simulink model "FBL_InvPD_RL"  (R2024b)
settings: Solver=VariableStepAuto  StartTime=0.0  StopTime=12  RelTol=1e-3
libraries: slpidlib x2, rllib x1
settings Model: Creator=shree  LastModifiedBy=shree

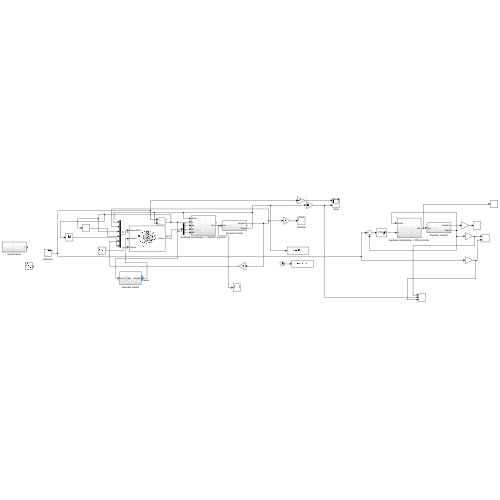
[thumbnail: Simulink's stored preview of the top-level diagram]
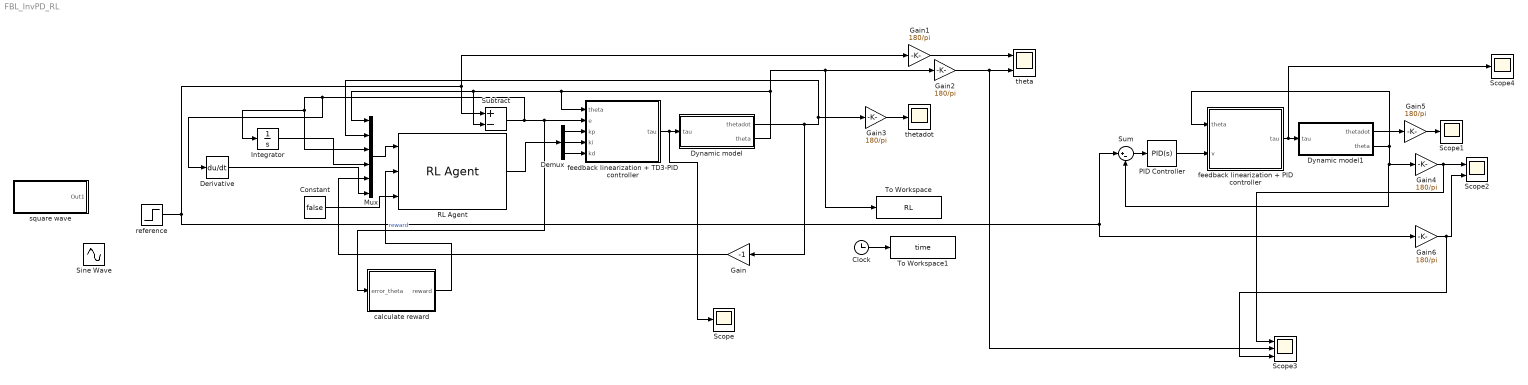
== system FBL_InvPD_RL ==
  Clock : Clock
  Constant : Constant  Value=false
  Demux : Demux  Outputs=3
  Derivative : Derivative
  Dynamic model : Subsystem
  Dynamic model1 : Subsystem
  Gain : Gain  Gain=-1
  Gain{1..6} (6 alike) : Gain  Gain=180/pi
  Integrator : Integrator
  Mux : Mux  Inputs=6
  PID Controller : slpidlib/PID Controller  Controller=PID  Form=Parallel  TimeDomain=Continuous-time  UseExternalTs=off  SampleTime=-1  IntegratorMethod=Forward Euler  FilterMethod=Forward Euler  ControllerParametersSource=internal  P=5.32832873411681  I=1.90556460171503  UseKiTs=off  D=3.52131946383864  UseExternalDerivativeSource=off  N=800  UseFilter=on  TunerSelectOption=Transfer Function Based (PID Tuner App)  InitialConditionSource=internal  InitialConditionForIntegrator=0  InitialConditionForFilter=0  DifferentiatorICPrevScaledInput=0  ExternalReset=none  TrackingMode=off  Kt=1  LimitOutput=on  SatLimitsSource=internal  UpperSaturationLimit=30  LowerSaturationLimit=-30  LinearizeAsGain=on  AntiWindupMode=none  Kb=1  LimitIntegrator=off  UpperIntegratorSaturationLimit=inf  LowerIntegratorSaturationLimit=-inf  POutMin=[]  POutMax=[]  IOutMin=[]  IOutMax=[]  DOutMin=[]  DOutMax=[]  NOutMin=[]  NOutMax=[]  SumOutMin=[]  SumOutMax=[]  SaturationOutMin=[]  SaturationOutMax=[]  PParamMin=[]  PParamMax=[]  IParamMin=[]  IParamMax=[]  DParamMin=[]  DParamMax=[]  NParamMin=[]  NParamMax=[]  KbParamMin=[]  KbParamMax=[]  KtParamMin=[]  KtParamMax=[]  KbOutMin=[]  KbOutMax=[]  KtOutMin=[]  KtOutMax=[]  IntegratorOutMin=[]  IntegratorOutMax=[]  FilterOutMin=[]  FilterOutMax=[]  SumI1OutMin=[]  SumI1OutMax=[]  SumI2OutMin=[]  SumI2OutMax=[]  SumI3OutMin=[]  SumI3OutMax=[]  SumI4OutMin=[]  SumI4OutMax=[]  SumDOutMin=[]  SumDOutMax=[]  DifferentiatorOutMin=[]  DifferentiatorOutMax=[]  FilterDiffOutCoefMin=[]  FilterDiffOutCoefMax=[]  ReciprocalOutMin=[]  ReciprocalOutMax=[]  SumDenOutMin=[]  SumDenOutMax=[]  SumNumOutMin=[]  SumNumOutMax=[]  DivideOutMin=[]  DivideOutMax=[]  UdiffTsProdOutMin=[]  UdiffTsProdOutMax=[]  NTsProdOutMin=[]  NTsProdOutMax=[]  UintegralTsProdOutMin=[]  UintegralTsProdOutMax=[]  UngainTsProdOutMin=[]  UngainTsProdOutMax=[]  ClampingZeroOutDataTypeStr=Inherit: Inherit via back propagation  ClampingZeroOutMin=[]  ClampingZeroOutMax=[]  FilterDenConstantOutDataTypeStr=Inherit: Inherit via back propagation  FilterDenConstantOutMin=[]  FilterDenConstantOutMax=[]  PCopyOutDataTypeStr=Inherit: Inherit via back propagation  PCopyOutMin=[]  PCopyOutMax=[]  NCopyOutDataTypeStr=Inherit: Inherit via back propagation  NCopyOutMin=[]  NCopyOutMax=[]  IntegratorContinuousStateAttributes=''  IntegratorStateMustResolveToSignalObject=off  IntegratorRTWStateStorageClass=Auto  FilterContinuousStateAttributes=''  FilterStateMustResolveToSignalObject=off  FilterRTWStateStorageClass=Auto  ParallelPVariant=InternalParameters  IdealPVariant=Disabled  IVariant=InternalParameters  DVariant=InternalParameters  IntegratorVariant=Continuous  SatVariant=Enabled  AWVariant=Passthrough  PCopyVariant=Disabled  TRVariant=Disabled  FdbkBlocksVariant=Forward  IdealPFdbkVariant=Disabled  SatFdbkVariant=Disabled  DerivativeFilterVariant=ContFilter  NVariant=InternalParameters  NCopyVariant=Disabled  FilterICVariant=InternalICsFilter  IntegratorICVariant=InternalICs  ExternalResetVariant=Disabled  TRSumVariant=Passthrough  SumFdbkVariant=Disabled  SumVariant=Sum_PID  TsampFilterVariant=InternalTs  TsampNgainVariant=Passthrough  TsampIntegralVariant=Disabled_SignalSpec  ExternalSaturationOutDataTypeStr=Inherit: Same as second input  DerivativeSourceVariant=ErrorSignal  PreIntVariant=InternalPreInt
  RL Agent : rllib/RL Agent  Agent=agent  ExternalActionAsInput=off  ProvideLastAction=off  ProvideCumRwd=off  TreatAsDirectFeedthrough=on  UseStrictObservationDataTypes=off
  Scope : Scope
  Scope1 : Scope
  Scope2 : Scope  NumInputPorts=2
  Scope3 : Scope  NumInputPorts=3
  Scope4 : Scope
  Sine Wave : Sin  Amplitude=pi/2  Frequency=3  SampleTime=0
  Subtract : Sum  Inputs=+-
  Sum : Sum  Inputs=|+-
  To Workspace : ToWorkspace  VariableName=RL  SaveFormat=Timeseries  SampleTime=-1
  To Workspace1 : ToWorkspace  VariableName=time  SaveFormat=Timeseries  SampleTime=-1
  calculate reward : Subsystem
  feedback linearization + PID controller : Subsystem
  feedback linearization + TD3-PID controller : Subsystem
  reference : Step  After=pi/2  SampleTime=0
  square wave : Subsystem
  theta : Scope  NumInputPorts=2
  thetadot : Scope
  wires:
  feedback linearization + TD3-PID controller/1(tau) -> Scope/1, Dynamic model/1(tau)
  Dynamic model/2(theta) -> Mux/1, Subtract/2, feedback linearization + TD3-PID controller/1(theta), To Workspace/1, Gain2/1
  Dynamic model/1(thetadot) -> Gain/1, Mux/2, Gain3/1
  Subtract/1 -> Derivative/1, Mux/3, Integrator/1, feedback linearization + TD3-PID controller/2(e), calculate reward/1(error_theta)
  RL Agent/1 -> Demux/1
  Demux/1 -> feedback linearization + TD3-PID controller/3(kp)
  Demux/2 -> feedback linearization + TD3-PID controller/4(ki)
  Demux/3 -> feedback linearization + TD3-PID controller/5(kd)
  Mux/1 -> RL Agent/1
  Gain/1 -> Mux/5
  Integrator/1 -> Mux/4
  Derivative/1 -> Mux/6
  calculate reward/1(reward) -> RL Agent/2  "reward"
  Constant/1 -> RL Agent/3
  Clock/1 -> To Workspace1/1
  Gain1/1 -> theta/1
  Gain2/1 -> Scope3/2, theta/2
  Gain3/1 -> thetadot/1
  feedback linearization + PID controller/1(tau) -> Scope4/1, Dynamic model1/1(tau)
  Dynamic model1/2(theta) -> feedback linearization + PID controller/1(theta), Gain4/1, Sum/2
  PID Controller/1 -> feedback linearization + PID controller/2(v)
  reference/1 -> Sum/1, Gain6/1, Subtract/1, Gain1/1
  Sum/1 -> PID Controller/1
  Dynamic model1/1(thetadot) -> Gain5/1
  Gain4/1 -> Scope3/1, Scope2/1
  Gain5/1 -> Scope1/1
  Gain6/1 -> Scope3/3, Scope2/2

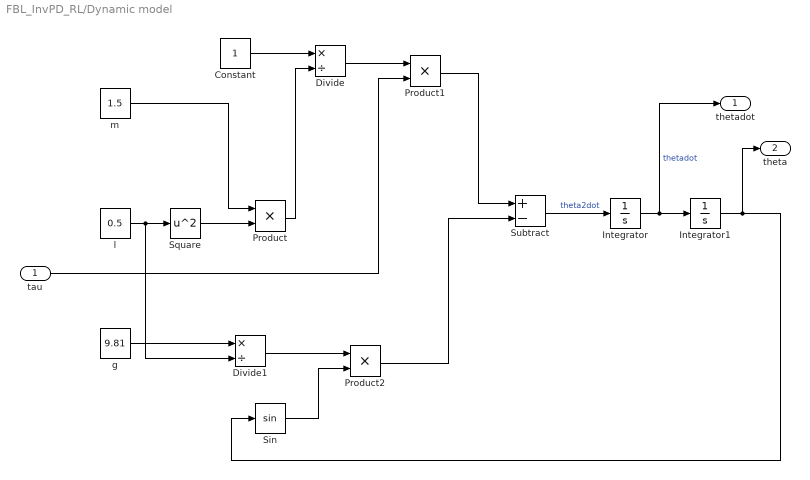
== system FBL_InvPD_RL/Dynamic model ==
  tau : Inport
  Constant : Constant
  Divide : Product  Inputs=*/
  Divide1 : Product  Inputs=*/
  Integrator : Integrator
  Integrator1 : Integrator
  Product : Product
  Product1 : Product
  Product2 : Product
  Sin : Trigonometry
  Square : Math  Operator=square
  Subtract : Sum  Inputs=+-
  g : Constant  Value=9.81
  l : Constant  Value=0.5
  m : Constant  Value=1.5
  thetadot : Outport
  theta : Outport  Port=2
  wires:
  Product2/1 -> Subtract/2
  Sin/1 -> Product2/2
  g/1 -> Divide1/1
  tau/1 -> Product1/2
  Constant/1 -> Divide/1
  l/1 -> Divide1/2, Square/1
  Divide1/1 -> Product2/1
  m/1 -> Product/1
  Divide/1 -> Product1/1
  Product1/1 -> Subtract/1
  Square/1 -> Product/2
  Subtract/1 -> Integrator/1  "theta2dot"
  Integrator1/1 -> theta/1, Sin/1
  Integrator/1 -> thetadot/1, Integrator1/1  "thetadot"
  Product/1 -> Divide/2

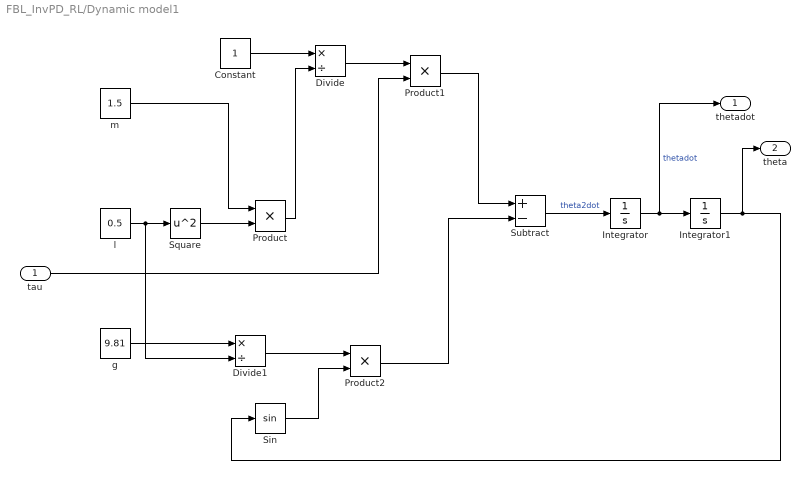
== system FBL_InvPD_RL/Dynamic model1 ==
  tau : Inport
  Constant : Constant
  Divide : Product  Inputs=*/
  Divide1 : Product  Inputs=*/
  Integrator : Integrator
  Integrator1 : Integrator
  Product : Product
  Product1 : Product
  Product2 : Product
  Sin : Trigonometry
  Square : Math  Operator=square
  Subtract : Sum  Inputs=+-
  g : Constant  Value=9.81
  l : Constant  Value=0.5
  m : Constant  Value=1.5
  thetadot : Outport
  theta : Outport  Port=2
  wires:
  Product2/1 -> Subtract/2
  Sin/1 -> Product2/2
  g/1 -> Divide1/1
  tau/1 -> Product1/2
  Constant/1 -> Divide/1
  l/1 -> Divide1/2, Square/1
  Divide1/1 -> Product2/1
  m/1 -> Product/1
  Divide/1 -> Product1/1
  Product1/1 -> Subtract/1
  Square/1 -> Product/2
  Subtract/1 -> Integrator/1  "theta2dot"
  Integrator1/1 -> theta/1, Sin/1
  Integrator/1 -> thetadot/1, Integrator1/1  "thetadot"
  Product/1 -> Divide/2

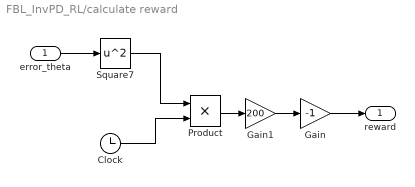
== system FBL_InvPD_RL/calculate reward ==
  error_theta : Inport
  Clock : Clock
  Gain : Gain  Gain=-1
  Gain1 : Gain  Gain=200
  Product : Product
  Square7 : Math  Operator=square
  reward : Outport
  wires:
  error_theta/1 -> Square7/1
  Square7/1 -> Product/1
  Clock/1 -> Product/2
  Product/1 -> Gain1/1
  Gain/1 -> reward/1
  Gain1/1 -> Gain/1

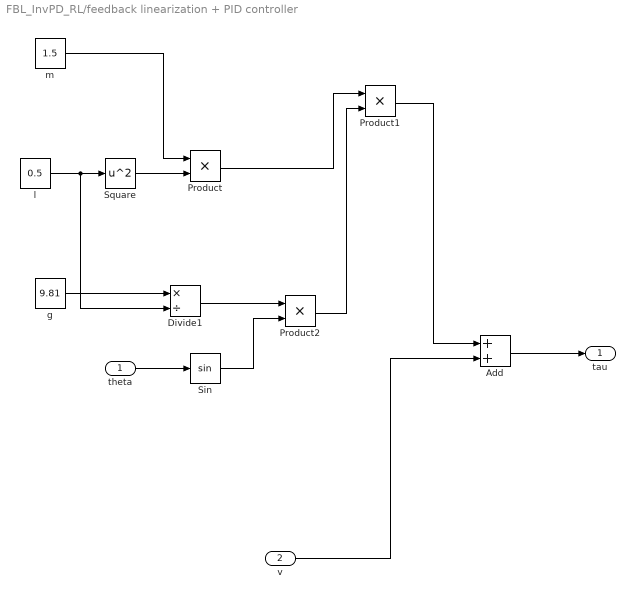
== system FBL_InvPD_RL/feedback linearization + PID controller ==
  theta : Inport
  v : Inport  Port=2
  Add : Sum
  Divide1 : Product  Inputs=*/
  Product : Product
  Product1 : Product
  Product2 : Product
  Sin : Trigonometry
  Square : Math  Operator=square
  g : Constant  Value=9.81
  l : Constant  Value=0.5
  m : Constant  Value=1.5
  tau : Outport
  wires:
  Product2/1 -> Product1/2
  Sin/1 -> Product2/2
  g/1 -> Divide1/1
  l/1 -> Divide1/2, Square/1
  Divide1/1 -> Product2/1
  m/1 -> Product/1
  Square/1 -> Product/2
  Product/1 -> Product1/1
  theta/1 -> Sin/1
  Product1/1 -> Add/1
  Add/1 -> tau/1
  v/1 -> Add/2

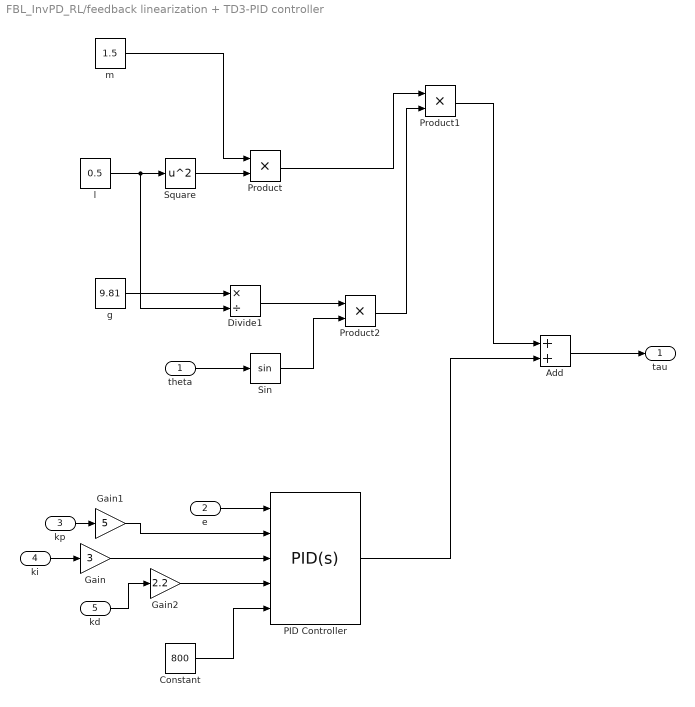
== system FBL_InvPD_RL/feedback linearization + TD3-PID controller ==
  theta : Inport
  e : Inport  Port=2
  kp : Inport  Port=3
  ki : Inport  Port=4
  kd : Inport  Port=5
  Add : Sum
  Constant : Constant  Value=800
  Divide1 : Product  Inputs=*/
  Gain : Gain  Gain=3
  Gain1 : Gain  Gain=5
  Gain2 : Gain  Gain=2.2
  PID Controller : slpidlib/PID Controller  Controller=PID  Form=Parallel  TimeDomain=Continuous-time  UseExternalTs=off  SampleTime=-1  IntegratorMethod=Forward Euler  FilterMethod=Forward Euler  ControllerParametersSource=external  P=1  I=1  UseKiTs=off  D=0  UseExternalDerivativeSource=off  N=100  UseFilter=on  TunerSelectOption=Transfer Function Based (PID Tuner App)  InitialConditionSource=internal  InitialConditionForIntegrator=0  InitialConditionForFilter=0  DifferentiatorICPrevScaledInput=0  ExternalReset=none  TrackingMode=off  Kt=1  LimitOutput=on  SatLimitsSource=internal  UpperSaturationLimit=30  LowerSaturationLimit=-30  LinearizeAsGain=on  AntiWindupMode=none  Kb=1  LimitIntegrator=off  UpperIntegratorSaturationLimit=inf  LowerIntegratorSaturationLimit=-inf  POutMin=[]  POutMax=[]  IOutMin=[]  IOutMax=[]  DOutMin=[]  DOutMax=[]  NOutMin=[]  NOutMax=[]  SumOutMin=[]  SumOutMax=[]  SaturationOutMin=[]  SaturationOutMax=[]  PParamMin=[]  PParamMax=[]  IParamMin=[]  IParamMax=[]  DParamMin=[]  DParamMax=[]  NParamMin=[]  NParamMax=[]  KbParamMin=[]  KbParamMax=[]  KtParamMin=[]  KtParamMax=[]  KbOutMin=[]  KbOutMax=[]  KtOutMin=[]  KtOutMax=[]  IntegratorOutMin=[]  IntegratorOutMax=[]  FilterOutMin=[]  FilterOutMax=[]  SumI1OutMin=[]  SumI1OutMax=[]  SumI2OutMin=[]  SumI2OutMax=[]  SumI3OutMin=[]  SumI3OutMax=[]  SumI4OutMin=[]  SumI4OutMax=[]  SumDOutMin=[]  SumDOutMax=[]  DifferentiatorOutMin=[]  DifferentiatorOutMax=[]  FilterDiffOutCoefMin=[]  FilterDiffOutCoefMax=[]  ReciprocalOutMin=[]  ReciprocalOutMax=[]  SumDenOutMin=[]  SumDenOutMax=[]  SumNumOutMin=[]  SumNumOutMax=[]  DivideOutMin=[]  DivideOutMax=[]  UdiffTsProdOutMin=[]  UdiffTsProdOutMax=[]  NTsProdOutMin=[]  NTsProdOutMax=[]  UintegralTsProdOutMin=[]  UintegralTsProdOutMax=[]  UngainTsProdOutMin=[]  UngainTsProdOutMax=[]  ClampingZeroOutDataTypeStr=Inherit: Inherit via back propagation  ClampingZeroOutMin=[]  ClampingZeroOutMax=[]  FilterDenConstantOutDataTypeStr=Inherit: Inherit via back propagation  FilterDenConstantOutMin=[]  FilterDenConstantOutMax=[]  PCopyOutDataTypeStr=Inherit: Inherit via back propagation  PCopyOutMin=[]  PCopyOutMax=[]  NCopyOutDataTypeStr=Inherit: Inherit via back propagation  NCopyOutMin=[]  NCopyOutMax=[]  IntegratorContinuousStateAttributes=''  IntegratorStateMustResolveToSignalObject=off  IntegratorRTWStateStorageClass=Auto  FilterContinuousStateAttributes=''  FilterStateMustResolveToSignalObject=off  FilterRTWStateStorageClass=Auto  ParallelPVariant=ExternalParameters  IdealPVariant=Disabled  IVariant=ExternalParameters  DVariant=ExternalParameters  IntegratorVariant=Continuous  SatVariant=Enabled  AWVariant=Passthrough  PCopyVariant=Disabled  TRVariant=Disabled  FdbkBlocksVariant=Forward  IdealPFdbkVariant=Disabled  SatFdbkVariant=Disabled  DerivativeFilterVariant=ContFilter  NVariant=ExternalParameters  NCopyVariant=Disabled  FilterICVariant=InternalICsFilter  IntegratorICVariant=InternalICs  ExternalResetVariant=Disabled  TRSumVariant=Passthrough  SumFdbkVariant=Disabled  SumVariant=Sum_PID  TsampFilterVariant=InternalTs  TsampNgainVariant=Passthrough  TsampIntegralVariant=Disabled_SignalSpec  ExternalSaturationOutDataTypeStr=Inherit: Same as second input  DerivativeSourceVariant=ErrorSignal  PreIntVariant=InternalPreInt
  Product : Product
  Product1 : Product
  Product2 : Product
  Sin : Trigonometry
  Square : Math  Operator=square
  g : Constant  Value=9.81
  l : Constant  Value=0.5
  m : Constant  Value=1.5
  tau : Outport
  wires:
  Product2/1 -> Product1/2
  Sin/1 -> Product2/2
  g/1 -> Divide1/1
  l/1 -> Divide1/2, Square/1
  Divide1/1 -> Product2/1
  m/1 -> Product/1
  Square/1 -> Product/2
  Product/1 -> Product1/1
  theta/1 -> Sin/1
  Product1/1 -> Add/1
  Add/1 -> tau/1
  PID Controller/1 -> Add/2
  e/1 -> PID Controller/1
  kp/1 -> Gain1/1
  ki/1 -> Gain/1
  Constant/1 -> PID Controller/5
  kd/1 -> Gain2/1
  Gain/1 -> PID Controller/3
  Gain1/1 -> PID Controller/2
  Gain2/1 -> PID Controller/4

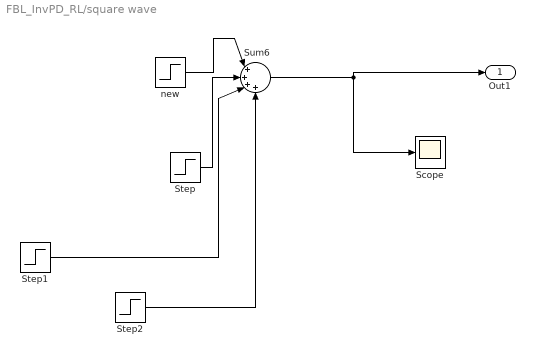
== system FBL_InvPD_RL/square wave ==
  Scope : Scope
  Step : Step  Time=4  SampleTime=0
  Step1 : Step  Time=8  After=-1  SampleTime=0
  Step2 : Step  Time=10  After=-1  SampleTime=0
  Sum6 : Sum  Inputs=|++++
  new : Step  Time=2  SampleTime=0.1
  Out1 : Outport
  wires:
  Sum6/1 -> Out1/1, Scope/1
  Step/1 -> Sum6/2
  new/1 -> Sum6/1
  Step1/1 -> Sum6/3
  Step2/1 -> Sum6/4
